simulink model "SFSPDiscreteSimulink"  (R2023b)
settings: Solver=VariableStepAuto  StartTime=0.0  StopTime=Tsim  RelTol=1e-3
values from neighbouring files (symbols this model uses):
  kc = (a1a-zc)/b0    [SFSPTuning.m]
  kr = (1-zc)/(a1a-zc)    [SFSPTuning.m]
  Ts = 0.25    [SFSPDiscrete.m]
undefined symbols (not defined in the file or in its folder): finaldisturbancevalue, finalnoisevalue, finalreferencevalue, initialdisturbancevalue, initialnoisevalue, initialreferencevalue, Tdisturbance, Tnoise, Tref
libraries: cstblocks x3
settings Model: Creator=klysm  LastModifiedBy=klysm

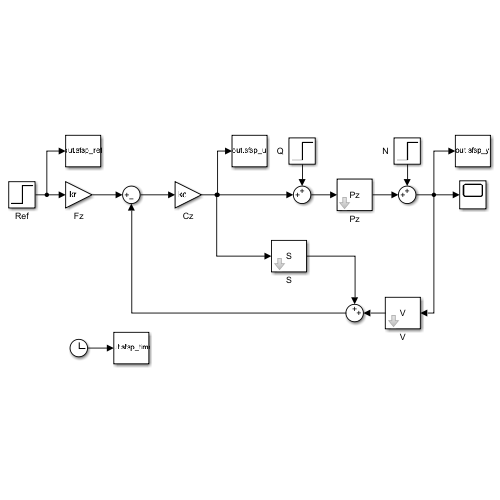
[thumbnail: Simulink's stored preview of the top-level diagram]
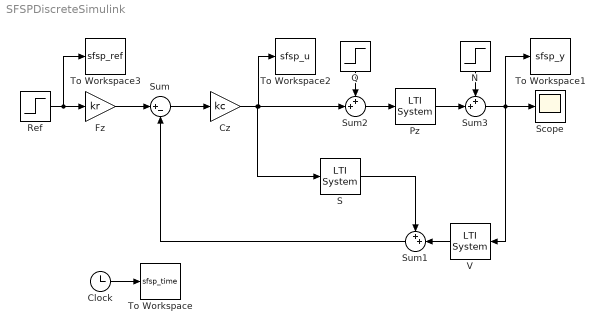
== system SFSPDiscreteSimulink ==
  Clock : Clock
  Cz : Gain  Gain=kc
  Fz : Gain  Gain=kr
  N : Step  Time=Tnoise  Before=initialnoisevalue  After=finalnoisevalue  SampleTime=Ts
  Pz : cstblocks/LTI System  sys=Pz  IC=[]  PadeOrder=0
  Q : Step  Time=Tdisturbance  Before=initialdisturbancevalue  After=finaldisturbancevalue  SampleTime=Ts
  Ref : Step  Time=Tref  Before=initialreferencevalue  After=finalreferencevalue  SampleTime=Ts
  S : cstblocks/LTI System  sys=S  IC=[]  PadeOrder=0
  Scope : Scope
  Sum : Sum  Inputs=|+-
  Sum1 : Sum  Inputs=++|
  Sum2 : Sum  Inputs=++|
  Sum3 : Sum  Inputs=++|
  To Workspace : ToWorkspace  VariableName=sfsp_time  SaveFormat=Timeseries  SampleTime=Ts
  To Workspace1 : ToWorkspace  VariableName=sfsp_y  SaveFormat=Timeseries  SampleTime=Ts
  To Workspace2 : ToWorkspace  VariableName=sfsp_u  SaveFormat=Timeseries  SampleTime=Ts
  To Workspace3 : ToWorkspace  VariableName=sfsp_ref  SaveFormat=Timeseries  SampleTime=Ts
  V : cstblocks/LTI System  sys=V  IC=[]  PadeOrder=0
  wires:
  Sum/1 -> Cz/1
  Fz/1 -> Sum/1
  V/1 -> Sum1/2
  S/1 -> Sum1/1
  Cz/1 -> To Workspace2/1, Sum2/2, S/1
  Ref/1 -> To Workspace3/1, Fz/1
  Sum1/1 -> Sum/2
  Sum2/1 -> Pz/1
  Q/1 -> Sum2/1
  Sum3/1 -> To Workspace1/1, Scope/1, V/1
  Clock/1 -> To Workspace/1
  Pz/1 -> Sum3/2
  N/1 -> Sum3/1
